simulink model "sim_topic4"  (R2023b)
settings: Solver=VariableStepAuto  StartTime=0.0  StopTime=N  RelTol=1e-3
undefined symbols (not defined in the file): denGdz, numGdz, T
settings Model: Creator=user  LastModifiedBy=user

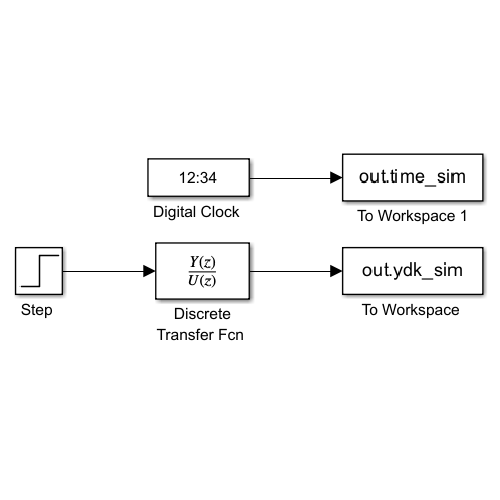
[thumbnail: Simulink's stored preview of the top-level diagram]
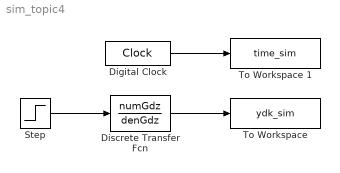
== system sim_topic4 ==
  "Digital Clock " : DigitalClock  SampleTime=T
  "Discrete Transfer Fcn " : DiscreteTransferFcn  Numerator=numGdz  Denominator=denGdz
  "Step " : Step  Time=0  SampleTime=T
  "To Workspace " : ToWorkspace  VariableName=ydk_sim  SampleTime=-1
  To Workspace 1 : ToWorkspace  VariableName=time_sim  SampleTime=-1
  wires:
  "Step "/1 -> "Discrete Transfer Fcn "/1
  "Discrete Transfer Fcn "/1 -> "To Workspace "/1
  "Digital Clock "/1 -> To Workspace 1/1
